simulink model "SLX07_addComponents"  (R2023a)
settings: Solver=VariableStepAuto  StartTime=0.0  StopTime=10  RelTol=1e-3
libraries: slpidlib x1
settings Model: NumberOfSteps=5  SnapshotBufferSize=50  SnapshotInterval=50  Creator=admin  LastModifiedBy=admin

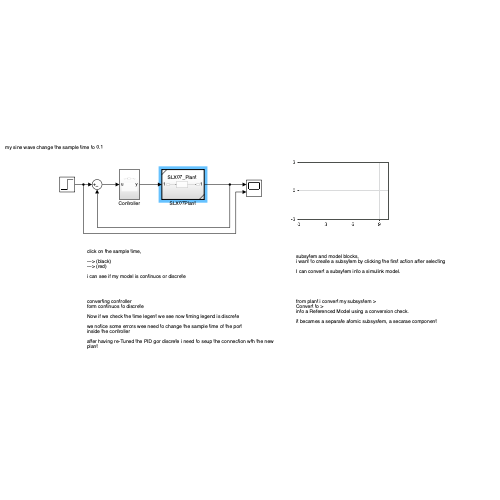
[thumbnail: Simulink's stored preview of the top-level diagram]
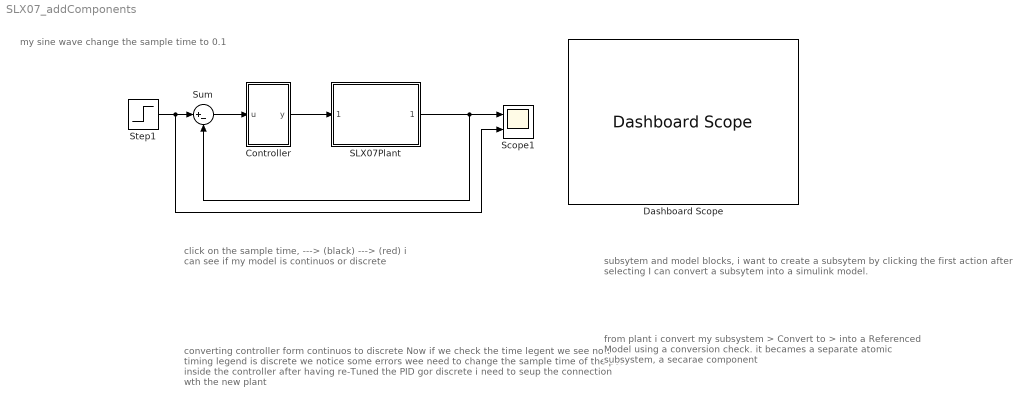
== system SLX07_addComponents ==
  note: my sine wave change the sample time to 0.1
  note: converting controller
      | form continuos to discrete
      |
      | Now if we check the time legent we see now timing legend is discrete
      |
      | we notice some errors wee need to change the sample time of the port
      | inside the controller
      |
      | after having re-Tuned the PID gor discrete i need to seup the connection wth the new plant
  note: click on the sample time,
      |
      | ---> (black)
      | ---> (red)
      |
      | i can see if my model is continuos or discrete
  note: from plant i convert my subsystem >
      | Convert to >
      | into a Referenced Model using a conversion check.
      |
      | it becames a separate atomic subsystem, a secarae component
  note: subsytem and model blocks,
      | i want to create a subsytem by clicking the first action after selecting
      |
      | I can convert a subsytem into a simulink model.
  Controller : Subsystem
  Dashboard Scope : DashboardScope
  SLX07Plant : Subsystem  TreatAsAtomicUnit=on  ReferencedSubsystem=SLX07_Plant
  Scope1 : Scope  NumInputPorts=2
  Step1 : Step  SampleTime=0.1
  Sum : Sum  Inputs=|+-
  wires:
  Step1/1 -> Sum/1, Scope1/2
  Sum/1 -> Controller/1(u)
  SLX07Plant/1 -> Sum/2, Scope1/1
  Controller/1(y) -> SLX07Plant/1

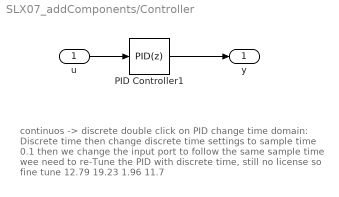
== system SLX07_addComponents/Controller ==
  note: continuos -> discrete
      | double click on PID
      | change time domain: Discrete time
      | then change discrete time settings to sample time 0.1
      |
      | then we change the input port to follow the same sample time
      |
      | wee need to re-Tune the PID with discrete time, still no license
      | so fine tune
      | 12.79
      | 19.23
      | 1.96
      | 11.7
  u : Inport  SampleTime=0.1
  PID Controller1 : slpidlib/PID Controller  Controller=PID  Form=Parallel  TimeDomain=Discrete-time  UseExternalTs=off  SampleTime=0.1  IntegratorMethod=Forward Euler  FilterMethod=Forward Euler  ControllerParametersSource=internal  P=13.79  I=19.23  UseKiTs=off  D=1.96  N=11.708  UseFilter=on  TunerSelectOption=Transfer Function Based (PID Tuner App)  InitialConditionSource=internal  InitialConditionForIntegrator=0  InitialConditionForFilter=0  DifferentiatorICPrevScaledInput=0  ExternalReset=none  TrackingMode=off  Kt=1  LimitOutput=off  SatLimitsSource=internal  UpperSaturationLimit=inf  LowerSaturationLimit=-inf  LinearizeAsGain=on  AntiWindupMode=none  Kb=1  LimitIntegrator=off  UpperIntegratorSaturationLimit=inf  LowerIntegratorSaturationLimit=-inf  POutMin=[]  POutMax=[]  IOutMin=[]  IOutMax=[]  DOutMin=[]  DOutMax=[]  NOutMin=[]  NOutMax=[]  SumOutMin=[]  SumOutMax=[]  SaturationOutMin=[]  SaturationOutMax=[]  PParamMin=[]  PParamMax=[]  IParamMin=[]  IParamMax=[]  DParamMin=[]  DParamMax=[]  NParamMin=[]  NParamMax=[]  KbParamMin=[]  KbParamMax=[]  KtParamMin=[]  KtParamMax=[]  KbOutMin=[]  KbOutMax=[]  KtOutMin=[]  KtOutMax=[]  IntegratorOutMin=[]  IntegratorOutMax=[]  FilterOutMin=[]  FilterOutMax=[]  SumI1OutMin=[]  SumI1OutMax=[]  SumI2OutMin=[]  SumI2OutMax=[]  SumI3OutMin=[]  SumI3OutMax=[]  SumI4OutMin=[]  SumI4OutMax=[]  SumDOutMin=[]  SumDOutMax=[]  DifferentiatorOutMin=[]  DifferentiatorOutMax=[]  FilterDiffOutCoefMin=[]  FilterDiffOutCoefMax=[]  ReciprocalOutMin=[]  ReciprocalOutMax=[]  SumDenOutMin=[]  SumDenOutMax=[]  SumNumOutMin=[]  SumNumOutMax=[]  DivideOutMin=[]  DivideOutMax=[]  UdiffTsProdOutMin=[]  UdiffTsProdOutMax=[]  NTsProdOutMin=[]  NTsProdOutMax=[]  UintegralTsProdOutMin=[]  UintegralTsProdOutMax=[]  UngainTsProdOutMin=[]  UngainTsProdOutMax=[]  ClampingZeroOutDataTypeStr=Inherit: Inherit via back propagation  ClampingZeroOutMin=[]  ClampingZeroOutMax=[]  FilterDenConstantOutDataTypeStr=Inherit: Inherit via back propagation  FilterDenConstantOutMin=[]  FilterDenConstantOutMax=[]  PCopyOutDataTypeStr=Inherit: Inherit via back propagation  PCopyOutMin=[]  PCopyOutMax=[]  NCopyOutDataTypeStr=Inherit: Inherit via back propagation  NCopyOutMin=[]  NCopyOutMax=[]  IntegratorContinuousStateAttributes=''  IntegratorStateMustResolveToSignalObject=off  IntegratorRTWStateStorageClass=Auto  FilterContinuousStateAttributes=''  FilterStateMustResolveToSignalObject=off  FilterRTWStateStorageClass=Auto  ParallelPVariant=InternalParameters  IdealPVariant=Disabled  IVariant=InternalParameters  DVariant=InternalParameters  IntegratorVariant=Discrete  SatVariant=Disabled  AWVariant=Passthrough  PCopyVariant=Disabled  TRVariant=Disabled  FdbkBlocksVariant=Forward  IdealPFdbkVariant=Disabled  SatFdbkVariant=Disabled  DerivativeFilterVariant=ForwardEulerFilter  NVariant=InternalParameters  NCopyVariant=Disabled  FilterICVariant=InternalICsFilter  IntegratorICVariant=InternalICs  ExternalResetVariant=Disabled  TRSumVariant=Passthrough  SumFdbkVariant=Disabled  SumVariant=Sum_PID  TsampFilterVariant=InternalTs  TsampNgainVariant=Passthrough  TsampIntegralVariant=Disabled_SignalSpec  ExternalSaturationOutDataTypeStr=Inherit: Same as second input
  y : Outport
  wires:
  PID Controller1/1 -> y/1
  u/1 -> PID Controller1/1
